simulink model "kulka_bb"  (R2015a)
settings: Solver=ode3  StartTime=0.0  StopTime=15  RelTol=1e-3
values from neighbouring files (symbols this model uses):
  d = 0.03    [skrypt.m]
  g = 9.8    [skrypt.m]
  J = 9.999e-6    (= 9.999e-06)    [skrypt.m]
  L = 1    [skrypt.m]
  m = 0.11    [skrypt.m]
  R = 0.015    [skrypt.m]
settings Model: Creator=Student  LastModifiedBy=lenovo

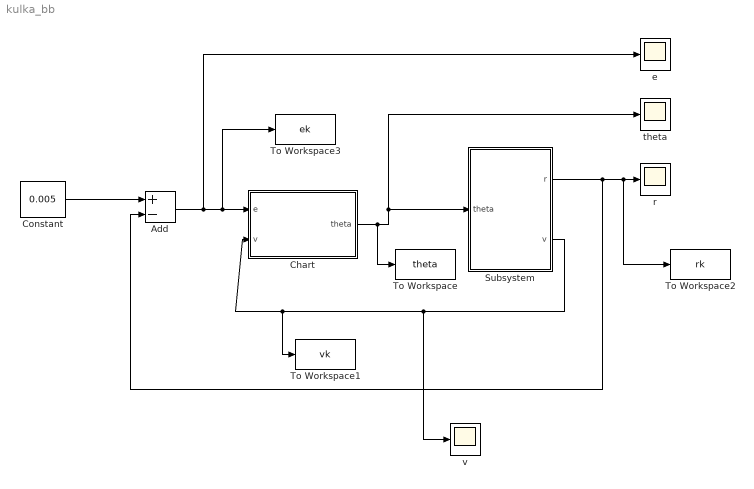
== system kulka_bb ==
  Add : Sum  Inputs=+-
  Chart : Stateflow chart  TreatAsAtomicUnit=on
  Constant : Constant  Value=0.005
  Subsystem : Subsystem
  To Workspace : ToWorkspace  VariableName=theta  SaveFormat=Timeseries  SampleTime=-1
  To Workspace1 : ToWorkspace  VariableName=vk  SaveFormat=Timeseries  SampleTime=-1
  To Workspace2 : ToWorkspace  VariableName=rk  SaveFormat=Timeseries  SampleTime=-1
  To Workspace3 : ToWorkspace  VariableName=ek  SaveFormat=Timeseries  SampleTime=-1
  e : Scope
      settings: SaveName=ScopeData2
  r : Scope
      settings: YMin=0  YMax=2.2e-06
  theta : Scope
      settings: YMin=-0.1  YMax=0.1
  v : Scope
      settings: SaveName=ScopeData3
  wires:
  Subsystem/1(r) -> Add/2, To Workspace2/1, r/1
  Constant/1 -> Add/1
  Chart/1(theta) -> To Workspace/1, theta/1, Subsystem/1(theta)
  Add/1 -> e/1, To Workspace3/1, Chart/1(e)
  Subsystem/2(v) -> v/1, To Workspace1/1, Chart/2(v)

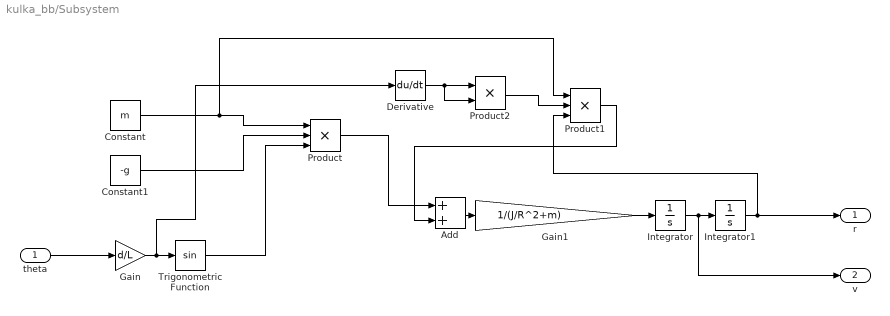
== system kulka_bb/Subsystem ==
  theta : Inport
  Add : Sum
  Constant : Constant  Value=m
  Constant1 : Constant  Value=-g
  Derivative : Derivative
  Gain : Gain  Gain=d/L
  Gain1 : Gain  Gain=1/(J/R^2+m)
  Integrator : Integrator
  Integrator1 : Integrator  LimitOutput=on  UpperSaturationLimit=1  LowerSaturationLimit=0
  Product : Product  Inputs=3
  Product1 : Product  Inputs=3
  Product2 : Product
  Trigonometric Function : Trigonometry
  r : Outport
  v : Outport  Port=2
  wires:
  Gain/1 -> Derivative/1, Trigonometric Function/1
  Integrator1/1 -> r/1, Product1/3
  Derivative/1 -> Product2/2, Product2/1
  Constant1/1 -> Product/2
  Trigonometric Function/1 -> Product/3
  Product/1 -> Add/1
  theta/1 -> Gain/1
  Constant/1 -> Product1/1, Product/1
  Integrator/1 -> v/1, Integrator1/1
  Add/1 -> Gain1/1
  Gain1/1 -> Integrator/1
  Product2/1 -> Product1/2
  Product1/1 -> Add/2

== stateflow chart kulka_bb/Chart ==
  state 1
    entry: theta=pi/64;
  state 2
    entry: theta=-pi/64;
  (default) -> 1
  1 -> 2 [order 2] : [v<=-0.001]
  1 -> 2 [order 1] : [e>=0]
  2 -> 1 [order 1] : [e<=0]
  2 -> 1 [order 2] : [v>=0.001]
  data: theta output; e input; v input
